simulink model "newss"  (Simulink 3.00)
settings: Solver=ode45  SolverMode=SingleTasking  StartTime=0.0  StopTime=20  MaxStep=0.010  RelTol=1e-3  AbsTol=1e-3
values from neighbouring files (symbols this model uses):
  du = dtu    [lambor.m]
  dy = dty    [lambor.m]    (also in paq.m = ny-1)
  nu = nu(2:5)    [lambor.m]
  ny = ny(2:5)    [lambor.m]    (also in paq.m = na)
  zh = input('Enter the upper limit for z:   ')    [data_newss.m]
  zl = input('Enter the lower limit for z:   ')    [data_newss.m]
  zsat = input('Enter saturation value for the magnitude of the state z:   ')    [data_newss.m]
  zsp = input('Enter desired set point for state z:   ')    [data_newss.m]
undefined symbols (not defined in the file or in its folder): cyi, czi, dhy, dhz, nhy, nhz
settings Model: TimeSaveName=t  SaveOutput=off

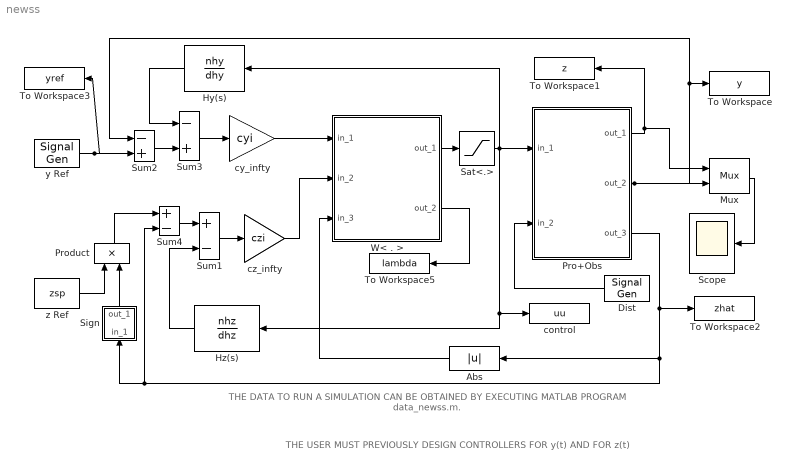
== system newss ==
  note: THE USER MUST PREVIOUSLY DESIGN CONTROLLERS FOR y(t) AND FOR z(t)
  note: THE DATA TO RUN A SIMULATION CAN BE OBTAINED
      |  BY EXECUTING  MATLAB PROGRAM data_newss.m.
  Abs : Abs  Orientation=left
  Dist : SignalGenerator  Orientation=left  WaveForm=square  Amplitude=1.000000  Frequency=0.200000  Units=rad/sec
  Hy(s) : TransferFcn  Orientation=left  Numerator=nhy  Denominator=dhy
      mask Type: HY
      mask Display: disp('Hy(s)')
  Hz(s) : TransferFcn  Orientation=left  Numerator=nhz  Denominator=dhz
      mask Type: HZ
      mask Display: disp('Hz(s)')
  Mux : Mux  Inputs=2
      settings: DisplayOption=none
  Pro+Obs : Subsystem
      mask Type: Proc. + Obs
      mask Display: disp('Proc.+Obs.')
  Product : Product  Orientation=up  Inputs=2  SaturateOnIntegerOverflow=on
  Sat<.> : Saturate  UpperLimit=zsat  LowerLimit=-zsat
  Scope : Scope
      settings: TickLabels=on  TimeRange=20.000000  YMin=-2.000000  YMax=2.000000  SaveToWorkspace=off  SaveName=ScopeData  DataFormat=Matrix
  Sign : Subsystem  Orientation=up
      mask Type: Sign
      mask Description: y = sign(x)
      mask Help: Sign Function:\n\t\t\ty = 1 if x > 0\n\t\t\ty = 0 if x = 0\n\t\t\ty = -1 if x < 0
      mask Display: plot(-50,-50,50,50,[-50,50],[0,0],[0,0],[-50,50],[-40,0],[-30,-30],[0,40],[30,30])
  Sum1 : Sum  Inputs=+-  SaturateOnIntegerOverflow=on
  Sum2 : Sum  Inputs=-+  SaturateOnIntegerOverflow=on
  Sum3 : Sum  Inputs=-+  SaturateOnIntegerOverflow=on
  Sum4 : Sum  Inputs=+-  SaturateOnIntegerOverflow=on
  To Workspace : ToWorkspace  VariableName=y  SampleTime=0  SaveFormat=Matrix
      settings: Buffer=10000
  To Workspace1 : ToWorkspace  VariableName=z  SampleTime=0  SaveFormat=Matrix
      settings: Buffer=10000
  To Workspace2 : ToWorkspace  VariableName=zhat  SampleTime=0  SaveFormat=Matrix
      settings: Buffer=10000
  To Workspace3 : ToWorkspace  VariableName=yref  SampleTime=0  SaveFormat=Matrix
      settings: Buffer=10000
  To Workspace5 : ToWorkspace  VariableName=lambda  SampleTime=0  SaveFormat=Matrix
      settings: Buffer=10000
  W< . > : Subsystem  mask(weighted switch){zlow=zl, zhigh=zh}
      mask help: weighted switch
      mask Display: disp('W. SWITCH')
  control : ToWorkspace  VariableName=uu  SampleTime=0  SaveFormat=Matrix
      settings: Buffer=10000
  cy_infty : Gain  Gain=cyi  SaturateOnIntegerOverflow=on
  cz_infty : Gain  Gain=czi  SaturateOnIntegerOverflow=on
  y Ref : SignalGenerator  WaveForm=square  Amplitude=1.000000  Frequency=0.300000  Units=rad/sec
  z Ref : Constant  Value=zsp
  wires:
  W< . >/1(out_1) -> Sat<.>/1
  cy_infty/1 -> W< . >/1(in_1)
  cz_infty/1 -> W< . >/2(in_2)
  Sum2/1 -> Sum3/2
  Sum3/1 -> cy_infty/1
  Sum4/1 -> Sum1/1
  Sum1/1 -> cz_infty/1
  Hy(s)/1 -> Sum3/1
  Hz(s)/1 -> Sum1/2
  Sign/1(out_1) -> Product/2
  z Ref/1 -> Product/1
  Product/1 -> Sum4/1
  Pro+Obs/3(out_3) -> To Workspace2/1, Sign/1(in_1), Sum4/2, Abs/1
  Mux/1 -> Scope/1
  Pro+Obs/1(out_1) -> To Workspace1/1, Mux/1
  Abs/1 -> W< . >/3(in_3)
  Sat<.>/1 -> Hy(s)/1, Pro+Obs/1(in_1), Hz(s)/1, control/1
  Pro+Obs/2(out_2) -> Sum2/1, To Workspace/1, Mux/2
  y Ref/1 -> Sum2/2, To Workspace3/1
  W< . >/2(out_2) -> To Workspace5/1
  Dist/1 -> Pro+Obs/2(in_2)

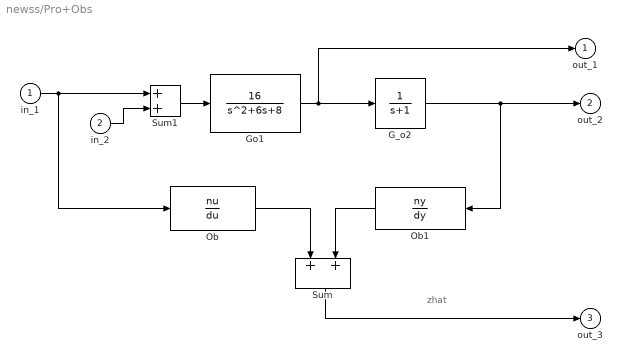
== system newss/Pro+Obs ==
  note: zhat
  in_1 : Inport  Port=1  PortWidth=-1  SampleTime=-1  DataType=auto
      settings: SignalType=auto
  in_2 : Inport  Port=2  PortWidth=-1  SampleTime=-1  DataType=auto
      settings: SignalType=auto
  G_o2 : TransferFcn  Numerator=[1]  Denominator=[1 1]
  Go1 : TransferFcn  Numerator=[16]  Denominator=[1 6 8]
  Ob : TransferFcn  Numerator=nu  Denominator=du
  Ob1 : TransferFcn  Orientation=left  Numerator=ny  Denominator=dy
  Sum : Sum  Orientation=down  Inputs=++  SaturateOnIntegerOverflow=on
  Sum1 : Sum  Inputs=++  SaturateOnIntegerOverflow=on
  out_1 : Outport  Port=1  InitialOutput=0
  out_2 : Outport  Port=2  InitialOutput=0
  out_3 : Outport  Port=3  InitialOutput=0
  wires:
  G_o2/1 -> out_2/1, Ob1/1
  Ob/1 -> Sum/1
  Ob1/1 -> Sum/2
  Sum1/1 -> Go1/1
  in_2/1 -> Sum1/2
  Sum/1 -> out_3/1
  Go1/1 -> G_o2/1, out_1/1
  in_1/1 -> Sum1/1, Ob/1

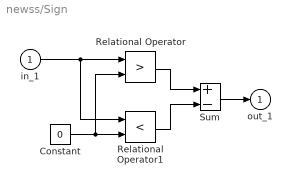
== system newss/Sign ==
  in_1 : Inport  Port=1  PortWidth=-1  SampleTime=-1  DataType=auto
      settings: SignalType=auto
  Constant : Constant  Value=0
  Relational Operator : RelationalOperator  Operator=>
  Relational Operator1 : RelationalOperator  Operator=<
  Sum : Sum  Inputs=+-  SaturateOnIntegerOverflow=on
  out_1 : Outport  Port=1  InitialOutput=0
  wires:
  in_1/1 -> Relational Operator/1, Relational Operator1/1
  Constant/1 -> Relational Operator1/2, Relational Operator/2
  Relational Operator1/1 -> Sum/2
  Relational Operator/1 -> Sum/1
  Sum/1 -> out_1/1

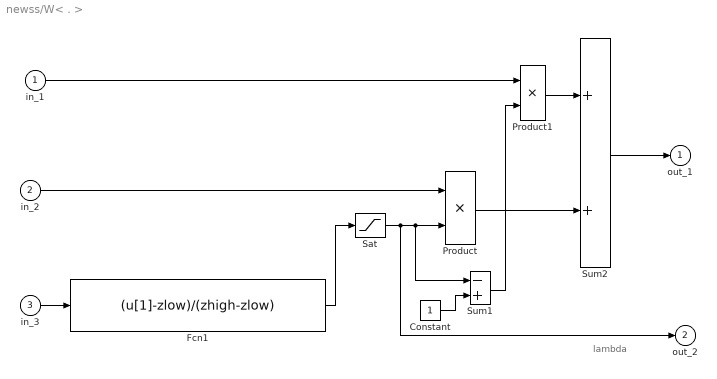
== system newss/W< . > ==
  note: lambda
  in_1 : Inport  Port=1  PortWidth=-1  SampleTime=-1  DataType=auto
      settings: SignalType=auto
  in_2 : Inport  Port=2  PortWidth=-1  SampleTime=-1  DataType=auto
      settings: SignalType=auto
  in_3 : Inport  Port=3  PortWidth=-1  SampleTime=-1  DataType=auto
      settings: SignalType=auto
  Constant : Constant  Value=1
  Fcn1 : Fcn  Expr=(u[1]-zlow)/(zhigh-zlow)
  Product : Product  Inputs=2  SaturateOnIntegerOverflow=on
  Product1 : Product  Inputs=2  SaturateOnIntegerOverflow=on
  Sat : Saturate  UpperLimit=1  LowerLimit=0
  Sum1 : Sum  Inputs=-+  SaturateOnIntegerOverflow=on
  Sum2 : Sum  Inputs=++  SaturateOnIntegerOverflow=on
  out_1 : Outport  Port=1  InitialOutput=0
  out_2 : Outport  Port=2  InitialOutput=0
  wires:
  Sum2/1 -> out_1/1
  Constant/1 -> Sum1/2
  in_2/1 -> Product/1
  Product/1 -> Sum2/2
  Product1/1 -> Sum2/1
  in_1/1 -> Product1/1
  in_3/1 -> Fcn1/1
  Fcn1/1 -> Sat/1
  Sum1/1 -> Product1/2
  Sat/1 -> Product/2, Sum1/1, out_2/1
